simulink model "problem8"  (R2020b)
settings: Solver=VariableStepAuto  StartTime=0.0  StopTime=10.0  RelTol=1e-3
model workspace (MAT data in the model file):
  OFF = Simulink.Parameter
  OFF.Value = 0
  OFF.DataType = 'auto'
  OFF.Dimensions = [1 1]
  ON = Simulink.Parameter
  ON.Value = 1
  ON.DataType = 'auto'
  ON.Dimensions = [1 1]
  Param = Simulink.Parameter
  Param.DataType = 'auto'
  Param.Dimensions = [0 0]
  Param1 = Simulink.Parameter
  Param1.DataType = 'auto'
  Param1.Dimensions = [0 0]
settings Model: Creator=k.Raviteja  LastModifiedBy=k.Raviteja

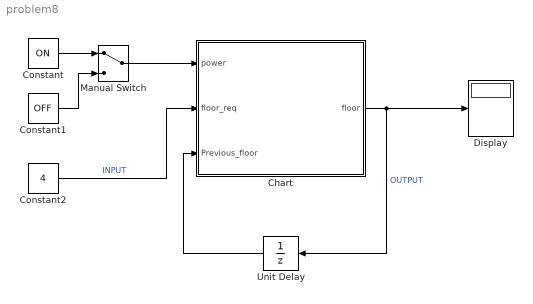
== system problem8 ==
  Chart : Stateflow chart  TreatAsAtomicUnit=on
  Constant : Constant  Value=ON
  Constant1 : Constant  Value=OFF
  Constant2 : Constant  Value=4
  Display : Display
  Manual Switch : ManualSwitch
  Unit Delay : UnitDelay  SampleTime=-1  HasFrameUpgradeWarning=on
  wires:
  Manual Switch/1 -> Chart/1(power)
  Chart/1(floor) -> Unit Delay/1, Display/1  "OUTPUT"
  Constant1/1 -> Manual Switch/2
  Constant/1 -> Manual Switch/1
  Constant2/1 -> Chart/2(floor_req)  "INPUT"
  Unit Delay/1 -> Chart/3(Previous_floor)

== stateflow chart problem8/Chart ==
  state LIFTON
    entry:
    floor=Previous_floor;
    state Requestedfloor
    state going_up
      entry:
      floor = floor + 1;
    state Going_down
      entry:
      floor = floor -1;
    (default) -> Requestedfloor
    going_up -> Requestedfloor [order 2] : [floor == floor_req]
    Going_down -> Requestedfloor [order 2] : [floor == floor_req]
    Requestedfloor -> going_up [order 1] : [floor < floor_req && floor_req<=5 ]
    Requestedfloor -> Going_down [order 2] : [floor > floor_req && floor_req>=0 ]
    Going_down -> Going_down [order 1] : [floor > floor_req]
    going_up -> going_up [order 1] : [floor < floor_req]
  state LIFTOFF
    entry:
    floor=Previous_floor;
  (default) -> LIFTOFF
  LIFTOFF -> LIFTON : [power == 1]
  LIFTON -> LIFTOFF : [power == 0]
  data: power input; floor output; floor_req input; Previous_floor input
